simulink library "plantModel"  (R2020a)
settings: Solver=VariableStepAuto  StartTime=0.0  StopTime=10.0  RelTol=1e-3
libraries: calcAeroLoadsInBdyFrame_cl x1, calcTangentialCoord_ul x1, calcGravForce_ul x1, makeOcB_cl x1, makeOcT_cl x1, sixDoFDynamics_cl x1
settings Model: Creator=Ayaz  LastModifiedBy=Ayaz

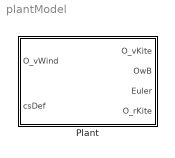
== system plantModel ==
  Plant : Subsystem  mask{mKite=36, jKite=eye(3), refArea=3, refSpan=5.5, refChord=0.55, gravAccl=9.81, rho=1.225, init_rKite=[0;0;-200], init_B_vKite=[0;0;0], init_Euler=[0;0;0], init_OwB=[0;0;0]}
      mask prompts: mKite "Kite mass [kg]"; jKite "Kite inertia matrix [kg*m^2]"; refArea "Reference wing area [m^2]"; refSpan "Reference wing span [m]"; refChord "Reference wing chord [m]"; gravAccl "Gravitational accleration [m/s^2]"; rho "Air density [kg/m^3]"; init_rKite "Kite initial inertial position [m]"; init_B_vKite "Kite initial body frame velocity [m/s]"; init_Euler "Kite initial Euler angles (roll,pithc,yaw) [rad]"; init_OwB "Kite initial angular velocity [rad/s]"
      mask TypeOptions mKite: sixDoFDynamics/mKite | gravForce/mKite
      mask TypeOptions jKite: sixDoFDynamics/jKite
      mask TypeOptions refArea: calcAeroLoads/refArea
      mask TypeOptions refSpan: calcAeroLoads/refSpan
      mask TypeOptions refChord: calcAeroLoads/refChord
      mask TypeOptions gravAccl: gravForce/gravAccl
      mask TypeOptions rho: calcAeroLoads/rho
      mask TypeOptions init_rKite: sixDoFDynamics/init_rKite
      mask TypeOptions init_B_vKite: sixDoFDynamics/init_B_vKite
      mask TypeOptions init_Euler: sixDoFDynamics/init_Euler
      mask TypeOptions init_OwB: sixDoFDynamics/init_OwB
      mask DialogControl ParameterGroupVar Prompt: Kite parameters
      mask DialogControl Container3 Prompt: Environment parameters
      mask DialogControl Container4 Prompt: Initial conditions

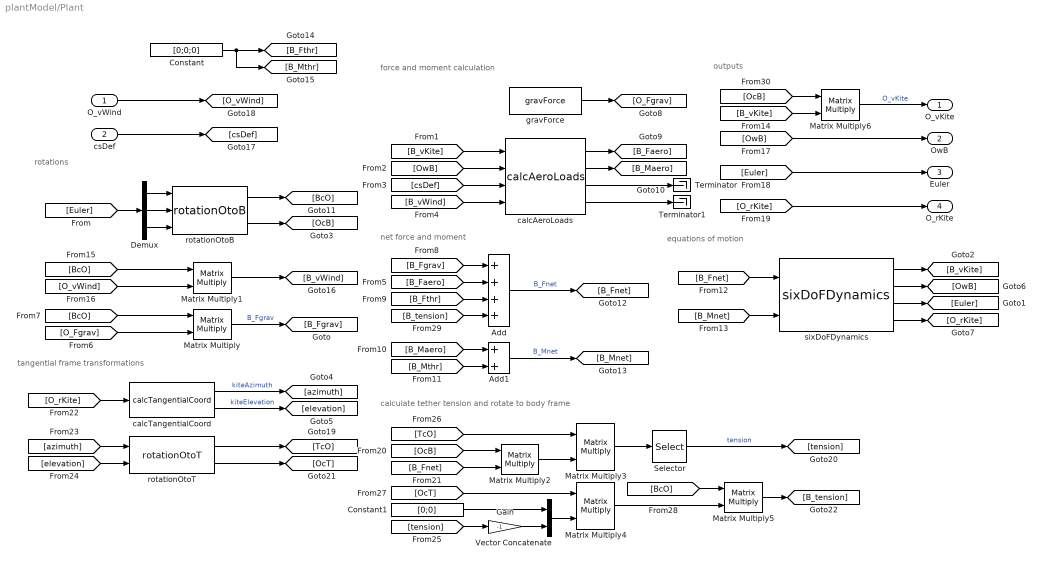
== system plantModel/Plant ==
  note: calculate tether tension and rotate to body frame
  note: tangential frame transformations
  note: equations of motion
  note: force and moment calculation
  note: rotations
  note: net force and moment
  note: outputs
  O_vWind : Inport
  csDef : Inport  Port=2
  Add : Sum  Inputs=++++
  Add1 : Sum
  Constant : Constant  Value=[0;0;0]  VectorParams1D=off
  Constant1 : Constant  Value=[0;0]  VectorParams1D=off
  Demux : Demux  Outputs=3
  Gain : Gain  Gain=-1
  Matrix Multiply{,1..6} (7 alike) : Product  Multiplication=Matrix(*)
  Selector : Selector  InputPortWidth=3  IndexOptions=Index vector (dialog)  Indices=3  OutputSizes=1
  Terminator : Terminator
  Terminator1 : Terminator
  Vector Concatenate : Concatenate
  calcAeroLoads : calcAeroLoadsInBdyFrame_cl/calcAeroLoads  refArea=refArea  refSpan=refSpan  refChord=refChord  rho=rho
  calcTangentialCoord : calcTangentialCoord_ul/calcTangentialCoord  SystemSampleTime=-1  Latency=0  AutoFrameSizeCalculation=off
  gravForce : calcGravForce_ul/gravForce  gravAccl=gravAccl  mKite=mKite
  rotationOtoB : makeOcB_cl/rotationOtoB  SystemSampleTime=-1  Latency=0  AutoFrameSizeCalculation=off
  rotationOtoT : makeOcT_cl/rotationOtoT  SystemSampleTime=-1  Latency=0  AutoFrameSizeCalculation=off
  sixDoFDynamics : sixDoFDynamics_cl/sixDoFDynamics  mKite=mKite  jKite=jKite  init_rKite=init_rKite  init_B_vKite=init_B_vKite  init_Euler=init_Euler  init_OwB=init_OwB
  O_vKite : Outport
  OwB : Outport  Port=2
  Euler : Outport  Port=3
  O_rKite : Outport  Port=4
  wires:
  sixDoFDynamics/3 -> [Euler]
  Demux/1 -> rotationOtoB/1
  Demux/2 -> rotationOtoB/2
  Demux/3 -> rotationOtoB/3
  [Euler] -> Demux/1
  sixDoFDynamics/1 -> [B_vKite]
  sixDoFDynamics/2 -> [OwB]
  sixDoFDynamics/4 -> [O_rKite]
  gravForce/1 -> [O_Fgrav]
  calcAeroLoads/1 -> [B_Faero]
  calcAeroLoads/2 -> [B_Maero]
  calcAeroLoads/3 -> Terminator/1
  calcAeroLoads/4 -> Terminator1/1
  [B_vKite] -> calcAeroLoads/1
  [OwB] -> calcAeroLoads/2
  [csDef] -> calcAeroLoads/3
  [B_vWind] -> calcAeroLoads/4
  rotationOtoB/1 -> [BcO]
  [BcO] -> Matrix Multiply/1
  [O_Fgrav] -> Matrix Multiply/2
  Matrix Multiply/1 -> [B_Fgrav]  "B_Fgrav"
  [B_Fgrav] -> Add/1
  [B_Faero] -> Add/2
  [B_Fthr] -> Add/3
  Add/1 -> [B_Fnet]  "B_Fnet"
  [B_Maero] -> Add1/1
  [B_Mthr] -> Add1/2
  Add1/1 -> [B_Mnet]  "B_Mnet"
  Constant/1 -> [B_Mthr], [B_Fthr]
  [B_Fnet] -> sixDoFDynamics/1
  [B_Mnet] -> sixDoFDynamics/2
  [BcO] -> Matrix Multiply1/1
  Matrix Multiply1/1 -> [B_vWind]
  [O_vWind] -> Matrix Multiply1/2
  O_vWind/1 -> [O_vWind]
  [O_rKite] -> O_rKite/1
  [OwB] -> OwB/1
  [Euler] -> Euler/1
  rotationOtoB/2 -> [OcB]
  csDef/1 -> [csDef]
  [OcB] -> Matrix Multiply2/1
  [B_Fnet] -> Matrix Multiply2/2
  [O_rKite] -> calcTangentialCoord/1
  calcTangentialCoord/1 -> [azimuth]  "kiteAzimuth"
  calcTangentialCoord/2 -> [elevation]  "kiteElevation"
  [azimuth] -> rotationOtoT/1
  [elevation] -> rotationOtoT/2
  rotationOtoT/1 -> [TcO]
  [TcO] -> Matrix Multiply3/1
  Matrix Multiply2/1 -> Matrix Multiply3/2
  Matrix Multiply3/1 -> Selector/1
  Selector/1 -> [tension]  "tension"
  [tension] -> Gain/1
  rotationOtoT/2 -> [OcT]
  Gain/1 -> Vector Concatenate/2
  Constant1/1 -> Vector Concatenate/1
  Vector Concatenate/1 -> Matrix Multiply4/2
  [OcT] -> Matrix Multiply4/1
  [BcO] -> Matrix Multiply5/1
  Matrix Multiply4/1 -> Matrix Multiply5/2
  Matrix Multiply5/1 -> [B_tension]
  [B_tension] -> Add/4
  [OcB] -> Matrix Multiply6/1
  [B_vKite] -> Matrix Multiply6/2
  Matrix Multiply6/1 -> O_vKite/1  "O_vKite"
